simulink library "LIB_TF_G_111"  (Simulink 8.6)
settings: Solver=ode45  StartTime=0.0  StopTime=10.0  RelTol=1e-3
PreLoadFcn:
  | if exist('tl_preloadfcn','file'), tl_preloadfcn(gcs,402); end
PostLoadFcn:
  | if exist('tl_postloadfcn','file'), tl_postloadfcn(gcs,402); end
undefined symbols (not defined in the file): ddv, u3, u4
libraries: tllib x1
(part 2 of 2)

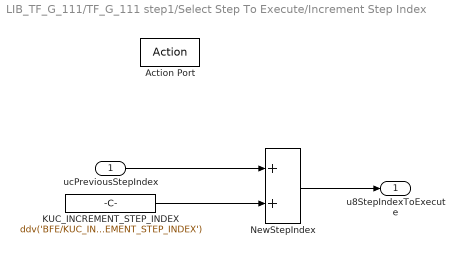
== system LIB_TF_G_111/TF_G_111 step1/Select Step To Execute/Increment Step Index ==
  ucPreviousStepIndex : Inport  RequirementInfo={} %GIDa_4cd58760_9ad1_4752_8fa3_fbb737a7480a  OutDataTypeStr=uint8
  Action Port : ActionPort  RequirementInfo="{}  %GIDa_54631830_eabe_46a1_add0_fae64ef8c3bc"
  KUC_INCREMENT_STEP_INDEX : Constant  RequirementInfo={} %GIDa_79068a5a_3d13_4a18_b0fc_31166480a7ba  Value=ddv('BFE/KUC_INCREMENT_STEP_INDEX')  OutDataTypeStr=Inherit: Inherit via back propagation  mask(TL_Constant){data={'output',{'variable','BFE/KUC_INCREMENT_STEP_INDEX'},'date',735951.66831914347}}
      settings: CopyFcn=if exist('tl_reset_reviewflag','file')==2,tl_reset_reviewflag(gcbh);end  DeleteFcn=if exist('delete_tlblock','file')==2,delete_tlblock(gcbh);end  NameChangeFcn=if exist('rename_tlblock','file')==2,rename_tlblock(gcbh);end  OpenFcn=if exist('tl_open_blockdlg','file')==2,tl_open_blockdlg(gcbh);else,open_system(gcbh,'parameter');end
      mask Help: eval(['if exist(''tl_online_help'',''file'') == 2, tl_online_help(''Topic'',''TL_Constant''),else, web([''jar:file:///'',matlabroot,''/help/toolbox/simulink/help.jar!/slref/' lower(get_param(gcbh,'Blocktype')) '.html''], ''-helpbrowser''),end'])
      mask Display: plot([-0.05, 1.05, NaN, -0.05, 1.05],[.01, .01, NaN, .99, .99])
  NewStepIndex : Sum  RequirementInfo={} %GIDa_df793995_a6cc_4c65_9ff1_a03c2377833c  OutDataTypeStr=Inherit: Inherit via back propagation  mask(TL_Sum){data={'output',{'name','u8NewStepIndex','type','UInt8'},'date',735951.66831876163}}
      settings: AttributesFormatString=Saturation: %<SaturateOnIntegerOverflow>  CopyFcn=if exist('tl_reset_reviewflag','file')==2,tl_reset_reviewflag(gcbh);end  DeleteFcn=if exist('delete_tlblock','file')==2,delete_tlblock(gcbh);end  NameChangeFcn=if exist('rename_tlblock','file')==2,rename_tlblock(gcbh);end  OpenFcn=if exist('tl_open_blockdlg','file')==2,tl_open_blockdlg(gcbh);else,open_system(gcbh,'parameter');end
      mask Help: eval(['if exist(''tl_online_help'',''file'') == 2, tl_online_help(''Topic'',''TL_Sum''),else, web([''jar:file:///'',matlabroot,''/help/toolbox/simulink/help.jar!/slref/' lower(get_param(gcbh,'Blocktype')) '.html''], ''-helpbrowser''),end'])
      mask Display: plot([-0.05, 1.05, NaN, -0.05, 1.05],[.01, .01, NaN, .99, .99])
  u8StepIndexToExecute : Outport  RequirementInfo={} %GIDa_6380abbd_d589_46e0_9418_0b26f4160665  InitialOutput=0
  wires:
  KUC_INCREMENT_STEP_INDEX/1 -> NewStepIndex/2
  ucPreviousStepIndex/1 -> NewStepIndex/1
  NewStepIndex/1 -> u8StepIndexToExecute/1

== system LIB_TF_G_111/TF_G_111 step1/Select Step To Execute/Init Step Id ==
  Action Port : ActionPort  RequirementInfo="{}  %GIDa_a1b0021c_7f73_45c2_aadd_b61db888fbe6"
  Constant : Constant  RequirementInfo={} %GIDa_7ece66ff_aed8_4357_a2d7_da4c23e09d80  Value=ddv('Common/KU8_ZERO')  OutDataTypeStr=uint8  mask(TL_Constant){data={'output',{'variable','Common/KU8_ZERO'},'autoscaling',{'mode',2,'scalingvalid',1},'date',735951.66831836803}}
      settings: CopyFcn=if exist('tl_reset_reviewflag','file')==2,tl_reset_reviewflag(gcbh);end  DeleteFcn=if exist('delete_tlblock','file')==2,delete_tlblock(gcbh);end  NameChangeFcn=if exist('rename_tlblock','file')==2,rename_tlblock(gcbh);end  OpenFcn=if exist('tl_open_blockdlg','file')==2,tl_open_blockdlg(gcbh);else,open_system(gcbh,'parameter');end
      mask Help: eval(['if exist(''tl_online_help'',''file'') == 2, tl_online_help(''Topic'',''TL_Constant''),else, web([''jar:file:///'',matlabroot,''/help/toolbox/simulink/help.jar!/slref/' lower(get_param(gcbh,'Blocktype')) '.html''], ''-helpbrowser''),end'])
      mask Display: plot([-0.05, 1.05, NaN, -0.05, 1.05],[.01, .01, NaN, .99, .99])
  u8StepIndexToExecute : Outport  RequirementInfo={} %GIDa_0b043a17_cf3e_4676_838c_da1c1d40acda  OutDataTypeStr=uint8  InitialOutput=0
  wires:
  Constant/1 -> u8StepIndexToExecute/1
